simulink model "Ass3Q2_4"  (R2018b)
settings: Solver=VariableStepAuto  StartTime=0.0  StopTime=40.0  RelTol=1e-3
values from neighbouring files (symbols this model uses):
  D = [X(3),0,c_0]    [Adaptive3.m]
  flag = 0    [Adaptive3.m]
undefined symbols (not defined in the file or in its folder): ss_mo, ss_pl
libraries: cstblocks x2
settings Model: Creator=bigfoot  LastModifiedBy=bigfoot

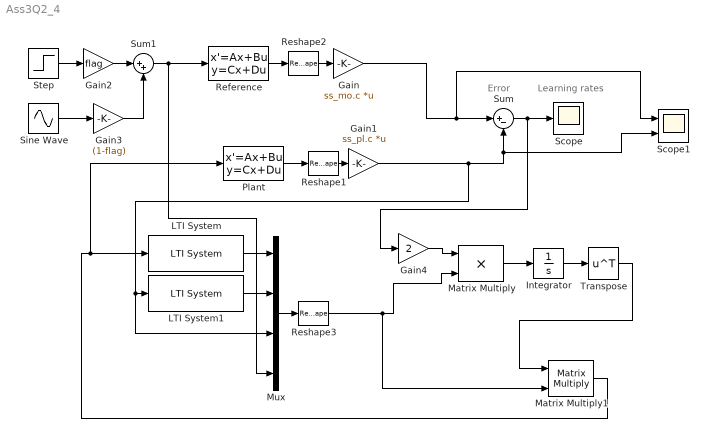
== system Ass3Q2_4 ==
  note: Learning rates
  note: Error
  Gain : Gain  Gain=ss_mo.c  Multiplication=Matrix(K*u)
  Gain1 : Gain  Gain=ss_pl.c  Multiplication=Matrix(K*u)
  Gain2 : Gain  Gain=flag
  Gain3 : Gain  Gain=(1-flag)
  Gain4 : Gain  Gain=2
  Integrator : Integrator
  LTI System : cstblocks/LTI System  sys=tf(1,[1 50])  IC=[]
  LTI System1 : cstblocks/LTI System  sys=tf(1,[1 50])  IC=[]
  Matrix Multiply : Product
  Matrix Multiply1 : Product  Multiplication=Matrix(*)
  Mux : Mux
  Plant : StateSpace  A=ss_pl.a  B=ss_pl.b  C=eye(2)  D=[0;0]  InitialCondition=[0,0]
  Reference : StateSpace  A=ss_mo.a  B=ss_mo.b  C=eye(2)  D=[0;0]  InitialCondition=0
  Reshape1 : Reshape  OutputDimensionality=Column vector (2-D)
  Reshape2 : Reshape  OutputDimensionality=Column vector (2-D)
  Reshape3 : Reshape  OutputDimensionality=Column vector (2-D)
  Scope : Scope
  Scope1 : Scope  NumInputPorts=2
  Sine Wave : Sin  SampleTime=0
  Step : Step  SampleTime=0
  Sum : Sum  Inputs=|+-
  Sum1 : Sum  Inputs=|++
  Transpose : Math  Operator=transpose  SaturateOnIntegerOverflow=on
  wires:
  Gain1/1 -> Mux/3, LTI System1/1, Scope1/2, Sum/2
  Gain/1 -> Scope1/1, Sum/1
  Sum/1 -> Gain4/1, Scope/1
  Sum1/1 -> Mux/4, Reference/1
  Reference/1 -> Reshape2/1
  Reshape2/1 -> Gain/1
  Plant/1 -> Reshape1/1
  Reshape1/1 -> Gain1/1
  Step/1 -> Gain2/1
  Gain2/1 -> Sum1/1
  Sine Wave/1 -> Gain3/1
  Gain3/1 -> Sum1/2
  Transpose/1 -> Matrix Multiply1/1
  Matrix Multiply/1 -> Integrator/1
  Reshape3/1 -> Matrix Multiply1/2, Matrix Multiply/2
  Gain4/1 -> Matrix Multiply/1
  Mux/1 -> Reshape3/1
  Integrator/1 -> Transpose/1
  Matrix Multiply1/1 -> Plant/1, LTI System/1
  LTI System/1 -> Mux/1
  LTI System1/1 -> Mux/2
